simulink model "Part4"  (R2019b)
settings: Solver=FixedStepAuto  StartTime=0.0  StopTime=60  FixedStep=0.1  RelTol=1e-3
model workspace (MAT data in the model file):
  A = 2.2
  Achsgetriebewirkungsgrad = 0.95
  E_ges = 60
  F_Reib = 40
  Getriebewirkungsgrad = 0.95
  M_gen_max = -2382
  MaxBremskraft = 7005.88
  Maxdrehmoment = 3460
  Pho = 1.225
  SOC_Init = 0.8
  c = 0.3
  eta1 = 0.95
  h = 0.5
  i_ag = 0.95
  i_g = 0.95
  l = 1.3
  lambda = 1.05
  miu = 1
  rdy = 0.34
values from neighbouring files (symbols this model uses):
  full_load_M_mot = [307.16713761 307.16713761 307.15125253 307.13548852 307.119845585 307.104323723 307.088922934 307.073643217 307.058484574 307.043447004 307.028530508 307.013735084 ... (79 elements, 1x79)]    [EBV_Par.mat]
  full_load_n = [0 200 400 600 800 1000 1200 1400 1600 1800 2000 2200 ... (79 elements, 1x79)]    [EBV_Par.mat]
  g = 9.81    [EBV_Par.mat]
  iag = 4    [EBV_Par.mat]
  ig = 3.12    [EBV_Par.mat]
  M_loss_mot_grid = [2.25037598951 2.25037598951 1.16187270775 0.818485589561 0.655488271287 0.566699700914 0.515063220158 0.480627768817 0.45851815067 0.444966043153 0.436284256227 0.436981398972 ... (2943 elements, 27x109)]    [EBV_Par.mat]
  M_lut = [0 2.86111111111 5.72222222222 8.58333333333 11.4444444444 14.3055555556 17.1666666667 20.0277777778 22.8888888889 25.75 28.6111111111 31.4722222222 ... (109 elements, 1x109)]    [EBV_Par.mat]
  n_lut = [0 615.384615385 1230.76923077 1846.15384615 2461.53846154 3076.92307692 3692.30769231 4307.69230769 4923.07692308 5538.46153846 6153.84615385 6769.23076923 ... (27 elements, 27x1)]    [EBV_Par.mat]
settings Model: Creator=kingtakepc  LastModifiedBy=kingtakepc
settings DebuggingCC: SFMachineParentedDataDiag=error

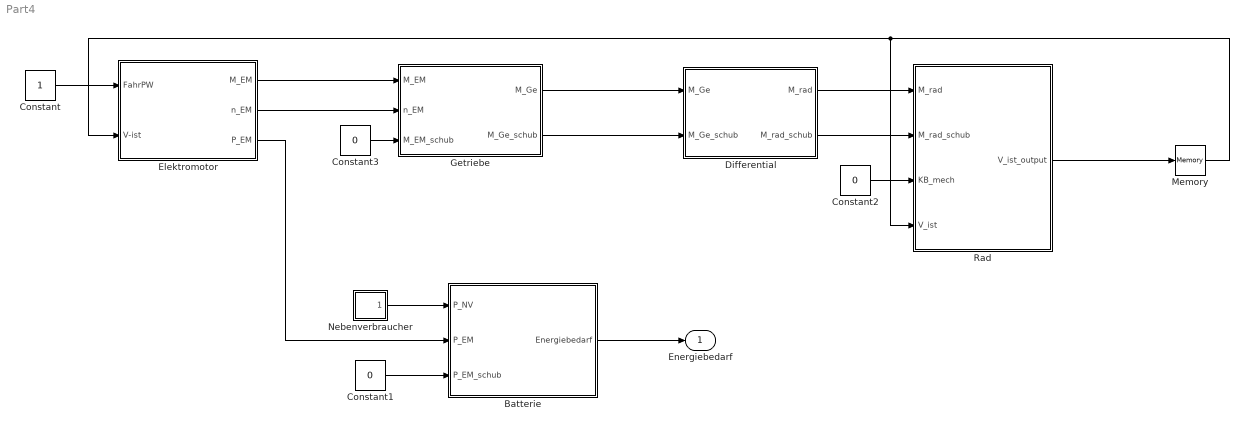
== system Part4 ==
  Batterie : Subsystem
  Constant : Constant
  Constant1 : Constant  Value=0
  Constant2 : Constant  Value=0
  Constant3 : Constant  Value=0
  Differential : Subsystem
  Elektromotor : Subsystem
  Getriebe : Subsystem
  Memory : Memory
  Nebenverbraucher : Subsystem
  Rad : Subsystem
  Energiebedarf : Outport
  wires:
  Getriebe/1(M_Ge) -> Differential/1(M_Ge)
  Differential/1(M_rad) -> Rad/1(M_rad)
  Nebenverbraucher/1(P_NV) -> Batterie/1(P_NV)
  Batterie/1(Energiebedarf) -> Energiebedarf/1
  Getriebe/2(M_Ge_schub) -> Differential/2(M_Ge_schub)
  Differential/2(M_rad_schub) -> Rad/2(M_rad_schub)
  Elektromotor/1(M_EM) -> Getriebe/1(M_EM)
  Elektromotor/2(n_EM) -> Getriebe/2(n_EM)
  Elektromotor/3(P_EM) -> Batterie/2(P_EM)
  Rad/1(V_ist_output) -> Memory/1
  Memory/1 -> Rad/4(V_ist), Elektromotor/2(V-ist)
  Constant/1 -> Elektromotor/1(FahrPW)
  Constant2/1 -> Rad/3(KB_mech)
  Constant3/1 -> Getriebe/3(M_EM_schub)
  Constant1/1 -> Batterie/3(P_EM_schub)

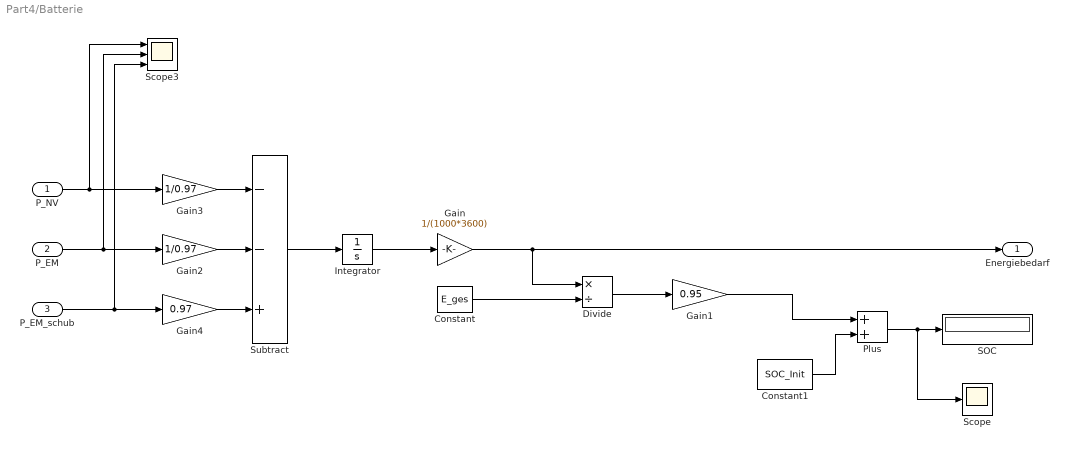
== system Part4/Batterie ==
  P_NV : Inport
  P_EM : Inport  Port=2
  P_EM_schub : Inport  Port=3
  Constant : Constant  Value=E_ges
  Constant1 : Constant  Value=SOC_Init
  Divide : Product  Inputs=*/
  Gain : Gain  Gain=1/(1000*3600)
  Gain1 : Gain  Gain=0.95
  Gain2 : Gain  Gain=1/0.97
  Gain3 : Gain  Gain=1/0.97
  Gain4 : Gain  Gain=0.97
  Integrator : Integrator
  Plus : Sum
  SOC : Display
  Scope : Scope
  Scope3 : Scope  NumInputPorts=3
  Subtract : Sum  Inputs=--+
  Energiebedarf : Outport
  wires:
  P_NV/1 -> Scope3/1, Gain3/1
  P_EM/1 -> Scope3/2, Gain2/1
  P_EM_schub/1 -> Scope3/3, Gain4/1
  Subtract/1 -> Integrator/1
  Integrator/1 -> Gain/1
  Gain/1 -> Divide/1, Energiebedarf/1
  Constant/1 -> Divide/2
  Divide/1 -> Gain1/1
  Constant1/1 -> Plus/2
  Gain2/1 -> Subtract/2
  Gain3/1 -> Subtract/1
  Gain4/1 -> Subtract/3
  Gain1/1 -> Plus/1
  Plus/1 -> Scope/1, SOC/1

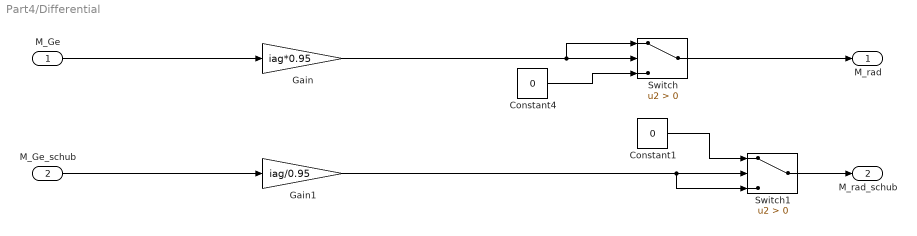
== system Part4/Differential ==
  M_Ge : Inport
  M_Ge_schub : Inport  Port=2
  Constant1 : Constant  Value=0
  Constant4 : Constant  Value=0
  Gain : Gain  Gain=iag*0.95
  Gain1 : Gain  Gain=iag/0.95
  Switch : Switch  Criteria=u2 > Threshold
  Switch1 : Switch  Criteria=u2 > Threshold
  M_rad : Outport
  M_rad_schub : Outport  Port=2
  wires:
  M_Ge/1 -> Gain/1
  M_Ge_schub/1 -> Gain1/1
  Switch/1 -> M_rad/1
  Gain/1 -> Switch/1, Switch/2
  Constant4/1 -> Switch/3
  Switch1/1 -> M_rad_schub/1
  Gain1/1 -> Switch1/3, Switch1/2
  Constant1/1 -> Switch1/1

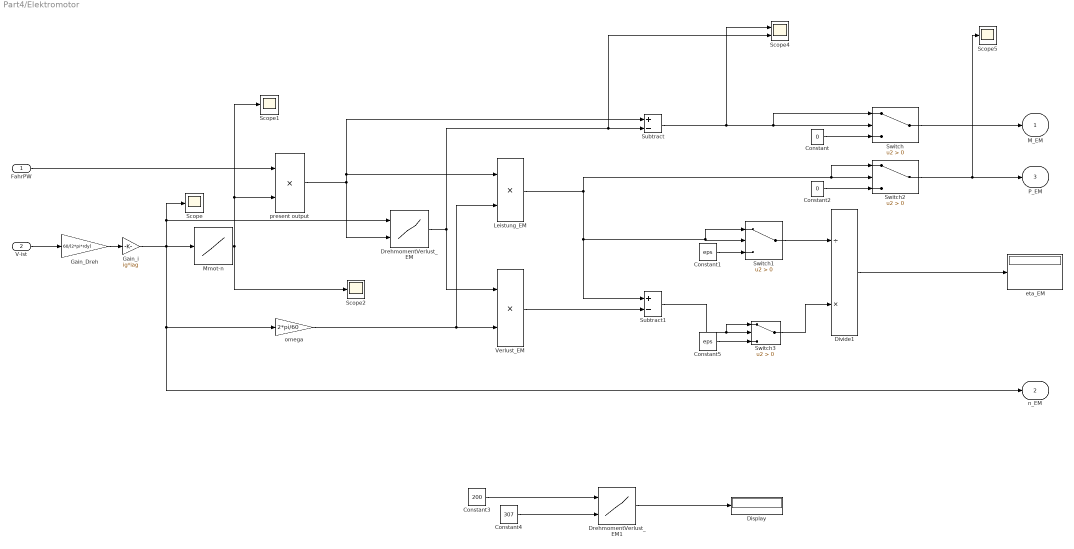
== system Part4/Elektromotor ==
  FahrPW : Inport
  V-ist : Inport  Port=2
  " Leistung_EM" : Product
  Constant : Constant  Value=0
  Constant1 : Constant  Value=eps
  Constant2 : Constant  Value=0
  Constant3 : Constant  Value=200
  Constant4 : Constant  Value=307
  Constant5 : Constant  Value=eps
  Display : Display
  Divide1 : Product  Inputs=/*
  DrehmomentVerlust_EM : Lookup_n-D  BreakpointsForDimension1=n_lut  BreakpointsForDimension2=M_lut  Table=M_loss_mot_grid  InternalRulePriority=Speed  RndMeth=Simplest  InputSameDT=on
  DrehmomentVerlust_EM1 : Lookup_n-D  BreakpointsForDimension1=n_lut  BreakpointsForDimension2=M_lut  Table=M_loss_mot_grid  InternalRulePriority=Speed  RndMeth=Simplest  InputSameDT=on
  Gain_Dreh : Gain  Gain=60/(2*pi*rdy)
  Gain_i : Gain  Gain=ig*iag
  Mmot-n : Lookup_n-D  NumberOfTableDimensions=1  BreakpointsForDimension1=full_load_n  Table=full_load_M_mot  InternalRulePriority=Speed  RndMeth=Simplest  InputSameDT=on
  Scope{,1..2,5} (4 alike) : Scope
  Scope4 : Scope  NumInputPorts=2
  Subtract : Sum  Inputs=+-
  Subtract1 : Sum  Inputs=+-
  Switch{,1..3} (4 alike) : Switch  Criteria=u2 > Threshold
  Verlust_EM : Product
  eta_EM : Display
  omega : Gain  Gain=2*pi/60
  present output : Product
  M_EM : Outport
  n_EM : Outport  Port=2
  P_EM : Outport  Port=3
  wires:
  FahrPW/1 -> present output/1
  V-ist/1 -> Gain_Dreh/1
  Gain_Dreh/1 -> Gain_i/1
  Gain_i/1 -> Scope/1, DrehmomentVerlust_EM/1, n_EM/1, omega/1, Mmot-n/1
  Mmot-n/1 -> Scope1/1, present output/2, Scope2/1
  DrehmomentVerlust_EM/1 -> Verlust_EM/1, Scope4/2, Subtract/2
  Subtract/1 -> Scope4/1, Switch/1, Switch/2
  Constant/1 -> Switch/3
  present output/1 -> DrehmomentVerlust_EM/2, Subtract/1, " Leistung_EM"/1
  omega/1 -> " Leistung_EM"/2, Verlust_EM/2
  " Leistung_EM"/1 -> Switch2/1, Switch2/2, Subtract1/1, Switch1/1, Switch1/2
  Switch1/1 -> Divide1/1
  Constant1/1 -> Switch1/3
  Divide1/1 -> eta_EM/1
  Constant2/1 -> Switch2/3
  Switch2/1 -> Scope5/1, P_EM/1
  Switch/1 -> M_EM/1
  Subtract1/1 -> Switch3/1, Switch3/2
  Verlust_EM/1 -> Subtract1/2
  Constant3/1 -> DrehmomentVerlust_EM1/1
  DrehmomentVerlust_EM1/1 -> Display/1
  Constant4/1 -> DrehmomentVerlust_EM1/2
  Constant5/1 -> Switch3/3
  Switch3/1 -> Divide1/2

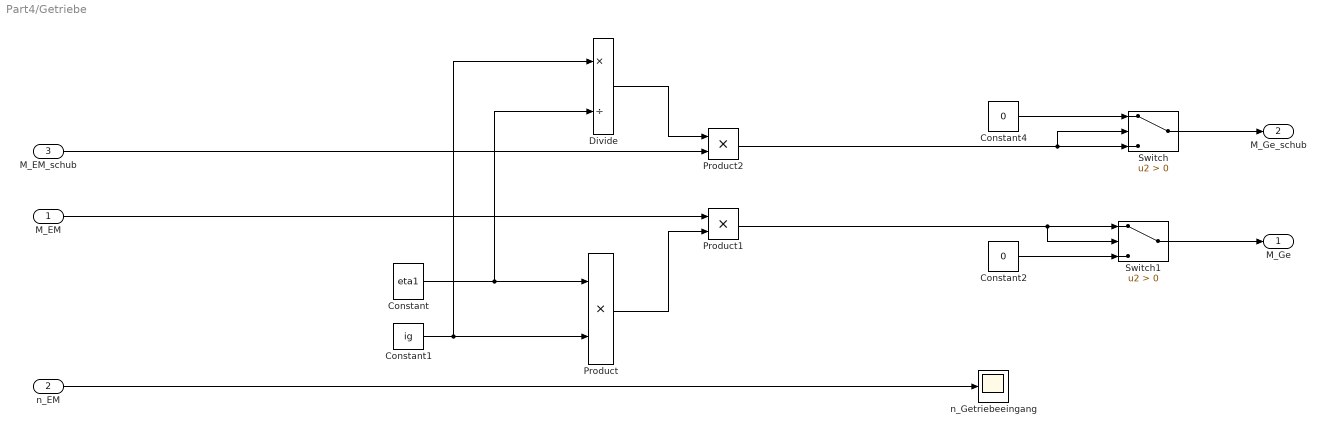
== system Part4/Getriebe ==
  M_EM : Inport
  n_EM : Inport  Port=2
  M_EM_schub : Inport  Port=3
  Constant : Constant  Value=eta1
  Constant1 : Constant  Value=ig
  Constant2 : Constant  Value=0
  Constant4 : Constant  Value=0
  Divide : Product  Inputs=*/
  Product : Product
  Product1 : Product
  Product2 : Product
  Switch : Switch  Criteria=u2 > Threshold
  Switch1 : Switch  Criteria=u2 > Threshold
  n_Getriebeeingang : Scope
  M_Ge : Outport
  M_Ge_schub : Outport  Port=2
  wires:
  Constant1/1 -> Divide/1, Product/2
  M_EM/1 -> Product1/1
  Constant/1 -> Divide/2, Product/1
  Product/1 -> Product1/2
  n_EM/1 -> n_Getriebeeingang/1
  M_EM_schub/1 -> Product2/2
  Divide/1 -> Product2/1
  Switch/1 -> M_Ge_schub/1
  Product2/1 -> Switch/2, Switch/3
  Constant4/1 -> Switch/1
  Switch1/1 -> M_Ge/1
  Product1/1 -> Switch1/2, Switch1/1
  Constant2/1 -> Switch1/3

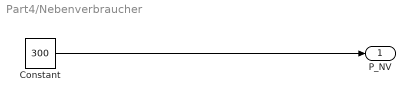
== system Part4/Nebenverbraucher ==
  Constant : Constant  Value=300
  P_NV : Outport
  wires:
  Constant/1 -> P_NV/1

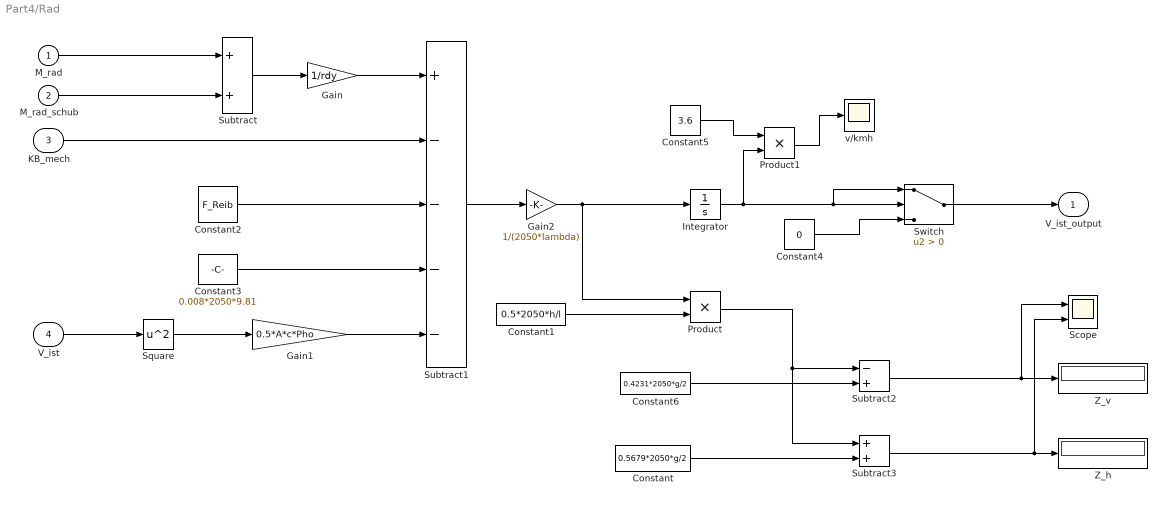
== system Part4/Rad ==
  M_rad : Inport
  M_rad_schub : Inport  Port=2
  KB_mech : Inport  Port=3
  V_ist : Inport  Port=4
  Constant : Constant  Value=0.5679*2050*g/2
  Constant1 : Constant  Value=0.5*2050*h/l
  Constant2 : Constant  Value=F_Reib
  Constant3 : Constant  Value=0.008*2050*9.81
  Constant4 : Constant  Value=0
  Constant5 : Constant  Value=3.6
  Constant6 : Constant  Value=0.4231*2050*g/2
  Gain : Gain  Gain=1/rdy
  Gain1 : Gain  Gain=0.5*A*c*Pho
  Gain2 : Gain  Gain=1/(2050*lambda)
  Integrator : Integrator
  Product : Product
  Product1 : Product
  Scope : Scope  NumInputPorts=2
  Square : Math  Operator=square  SaturateOnIntegerOverflow=on
  Subtract : Sum
  Subtract1 : Sum  Inputs=+----
  Subtract2 : Sum  Inputs=-+
  Subtract3 : Sum
  Switch : Switch  Criteria=u2 > Threshold
  Z_h : Display
  Z_v : Display
  v/kmh : Scope
  V_ist_output : Outport
  wires:
  M_rad/1 -> Subtract/1
  M_rad_schub/1 -> Subtract/2
  Subtract/1 -> Gain/1
  Gain/1 -> Subtract1/1
  KB_mech/1 -> Subtract1/2
  Constant2/1 -> Subtract1/3
  Constant3/1 -> Subtract1/4
  V_ist/1 -> Square/1
  Square/1 -> Gain1/1
  Gain1/1 -> Subtract1/5
  Subtract1/1 -> Gain2/1
  Gain2/1 -> Product/1, Integrator/1
  Integrator/1 -> Product1/2, Switch/1, Switch/2
  Constant1/1 -> Product/2
  Subtract2/1 -> Scope/1, Z_v/1
  Subtract3/1 -> Scope/2, Z_h/1
  Product/1 -> Subtract3/1, Subtract2/1
  Constant/1 -> Subtract3/2
  Constant4/1 -> Switch/3
  Switch/1 -> V_ist_output/1
  Constant5/1 -> Product1/1
  Product1/1 -> v/kmh/1
  Constant6/1 -> Subtract2/2
